simulink library "xpcmeasurementcomputinglib"  (Simulink 6.0)
settings: Solver=ode45  SolverMode=SingleTasking  StartTime=0.0  StopTime=10.0  RelTol=1e-3
undefined symbols (not defined in the file or in its folder): madcbciodas, madcbpcidas, madcbpcidas1600, mctr05checks, mdacbisa, mdacbpcidas, mdacbpcidas1600, mdacbpcidda0x12, mdiocbpcipdisox, menccbcioquadcount, misa8255, mpci8255, mtccb
libraries: xpcmeasurementcomputinglib x18
(part 4 of 4)

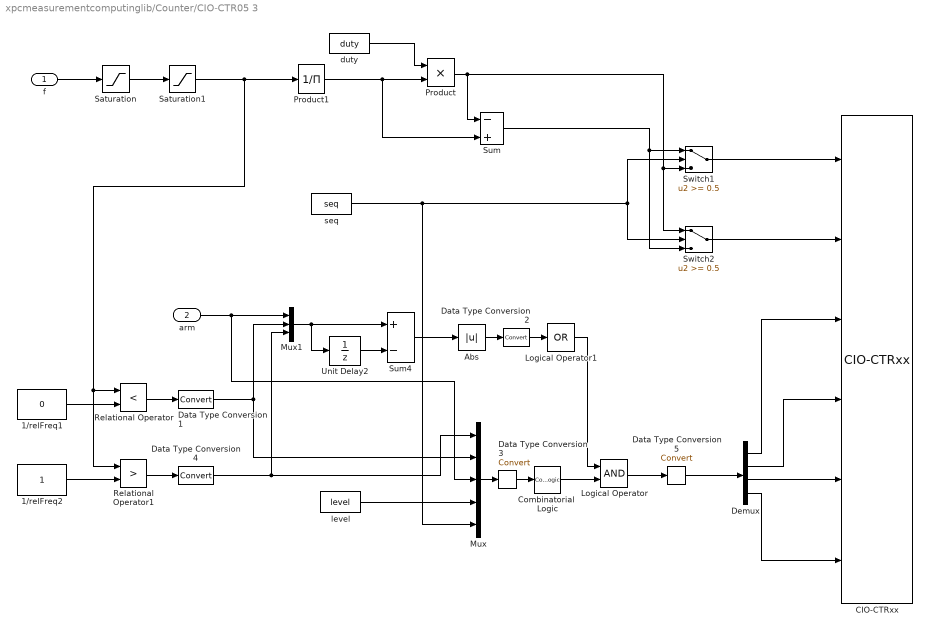
== system xpcmeasurementcomputinglib/Counter/CIO-CTR05 3 ==
  f : Inport  LatchInput=off
  arm : Inport  Port=2  LatchInput=off
  1/relFreq1 : Constant  Value=0
  1/relFreq2 : Constant
  Abs : Abs  SaturateOnIntegerOverflow=on
  "CIO-CTRxx " : xpcmeasurementcomputinglib/Counter/CIO-CTRxx   mastermode=MasterMode  countermode=CounterMode  init=Init  commands=Runtime  term=Term  ts=Ts  baseAddress=baseAddress
  Combinatorial  Logic : CombinatorialLogic  TruthTable=[0,0,1,0;0,0,1,0;0,0,0,1;0,0,0,1;0,1,0,0;1,0,0,0;0,1,0,0;1,0,0,0;0,0,1,0;0,0,1,0;0,0,0,1;0,0,0,1;0,0,1,0;0,0,1,0;0,0,1,0;0,0,1,0;0,0,1,0;0,0,1,0;0,0,0,1;0,0,0,1;0,0,0,1;0,0,0,1;0,0,0,1;0,0,0,1;0,0,0,0;0,0,0,0;0,0,0,0;0,0,0,0;0,0,0,0;0,0,0,0;0,0,0,0;0,0,0,0]
  Data Type Conversion1 : DataTypeConversion  OutDataTypeMode=double  SaturateOnIntegerOverflow=on  RndMeth=Zero
  Data Type Conversion2 : DataTypeConversion  SaturateOnIntegerOverflow=on  RndMeth=Zero
  Data Type Conversion3 : DataTypeConversion  SaturateOnIntegerOverflow=on  RndMeth=Zero
  Data Type Conversion4 : DataTypeConversion  OutDataTypeMode=double  SaturateOnIntegerOverflow=on  RndMeth=Zero
  Data Type Conversion5 : DataTypeConversion  SaturateOnIntegerOverflow=on  RndMeth=Zero
  Demux : Demux
  Logical Operator : Logic
  Logical Operator1 : Logic  Operator=OR  Inputs=1
  Mux : Mux  Inputs=5
  Mux1 : Mux  Inputs=3
  Product : Product  SaturateOnIntegerOverflow=on  InputSameDT=on
  Product1 : Product  Inputs=/  SaturateOnIntegerOverflow=on  InputSameDT=on
  Relational Operator : RelationalOperator  Operator=<  InputSameDT=on
  Relational Operator1 : RelationalOperator  Operator=>  InputSameDT=on
  Saturation : Saturate  UpperLimit=duty/2  LowerLimit=duty/(2^16-1)  ZeroCross=off
  Saturation1 : Saturate  UpperLimit=(1-duty)/2  LowerLimit=(1-duty)/(2^16-1)  ZeroCross=off
  Sum : Sum  Inputs=-+  SaturateOnIntegerOverflow=on  InputSameDT=on
  Sum4 : Sum  Inputs=+-  SaturateOnIntegerOverflow=on  InputSameDT=on
  Switch1 : Switch  Threshold=0.5  InputSameDT=on
  Switch2 : Switch  Threshold=0.5  InputSameDT=on
  Unit Delay2 : UnitDelay  X0=2  SampleTime=Ts
  duty : Constant  Value=duty
  level : Constant  Value=level
  seq : Constant  Value=seq
  wires:
  Data Type Conversion5/1 -> Demux/1
  Data Type Conversion3/1 -> Combinatorial  Logic/1
  Data Type Conversion2/1 -> Logical Operator1/1
  Data Type Conversion1/1 -> Mux1/2, Mux/2
  Data Type Conversion4/1 -> Mux1/3, Mux/1
  1/relFreq1/1 -> Relational Operator/2
  Product/1 -> Sum/1, Switch1/3, Switch2/1
  1/relFreq2/1 -> Relational Operator1/2
  Relational Operator1/1 -> Data Type Conversion4/1
  Relational Operator/1 -> Data Type Conversion1/1
  Combinatorial  Logic/1 -> Logical Operator/2
  Logical Operator/1 -> Data Type Conversion5/1
  Unit Delay2/1 -> Sum4/2
  Sum4/1 -> Abs/1
  Logical Operator1/1 -> Logical Operator/1
  Demux/1 -> "CIO-CTRxx "/3
  Demux/2 -> "CIO-CTRxx "/4
  Demux/3 -> "CIO-CTRxx "/5
  Demux/4 -> "CIO-CTRxx "/6
  level/1 -> Mux/4
  Switch1/1 -> "CIO-CTRxx "/1
  Switch2/1 -> "CIO-CTRxx "/2
  seq/1 -> Switch1/2, Switch2/2, Mux/5
  Sum/1 -> Switch1/1, Switch2/3
  Saturation/1 -> Saturation1/1
  f/1 -> Saturation/1
  Mux1/1 -> Sum4/1, Unit Delay2/1
  arm/1 -> Mux1/1, Mux/3
  Abs/1 -> Data Type Conversion2/1
  Mux/1 -> Data Type Conversion3/1
  Saturation1/1 -> Product1/1, Relational Operator1/1, Relational Operator/1
  duty/1 -> Product/1
  Product1/1 -> Product/2, Sum/2

== system xpcmeasurementcomputinglib/Counter/CIO-CTR05 4 ==
  "CIO-CTRxx " : xpcmeasurementcomputinglib/Counter/CIO-CTRxx   mastermode=MasterMode  countermode=CounterMode  init=Init  commands=Runtime  term=Term  ts=Ts  baseAddress=baseAddress
  Demux : Demux  Outputs=2
  Product : Product  Inputs=/  SaturateOnIntegerOverflow=on  InputSameDT=on
  Product1 : Product  Inputs=**  SaturateOnIntegerOverflow=on  InputSameDT=on
  f : Outport
  dc : Outport  Port=2
  wires:
  Product1/1 -> dc/1
  Product/1 -> Product1/2, f/1
  Demux/2 -> Product/1
  Demux/1 -> Product1/1
  "CIO-CTRxx "/1 -> Demux/1

== system xpcmeasurementcomputinglib/Counter/CIO-CTR05 5 ==
  "CIO-CTRxx " : xpcmeasurementcomputinglib/Counter/CIO-CTRxx   mastermode=MasterMode  countermode=CounterMode  init=Init  commands=Runtime  term=Term  ts=Ts  baseAddress=baseAddress
  Product : Product  Inputs=/  SaturateOnIntegerOverflow=on  InputSameDT=on
  f : Outport
  wires:
  Product/1 -> f/1
  "CIO-CTRxx "/1 -> Product/1

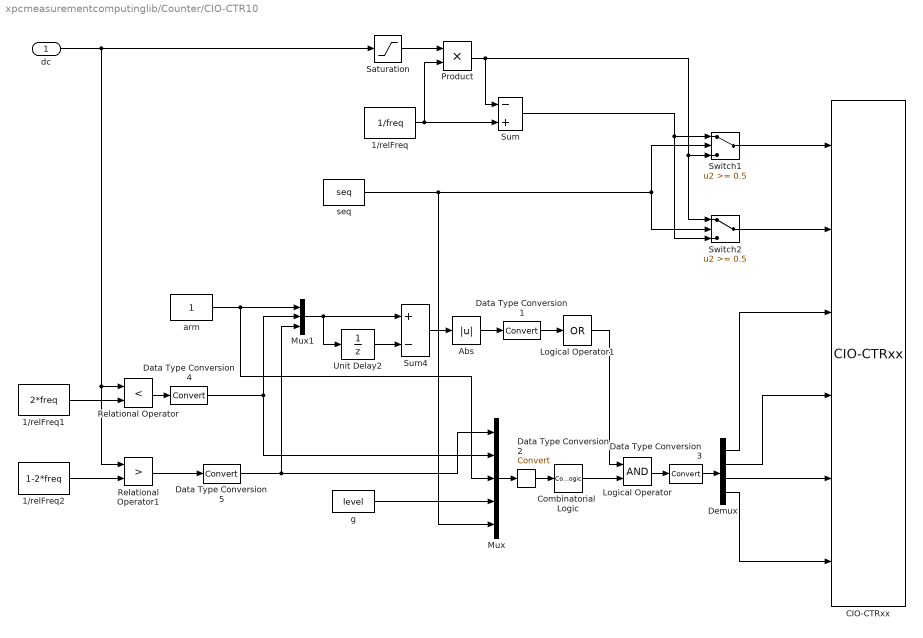
== system xpcmeasurementcomputinglib/Counter/CIO-CTR10  ==
  dc : Inport  LatchInput=off
  1/relFreq : Constant  Value=1/freq
  1/relFreq1 : Constant  Value=2*freq
  1/relFreq2 : Constant  Value=1-2*freq
  Abs : Abs  SaturateOnIntegerOverflow=on
  "CIO-CTRxx " : xpcmeasurementcomputinglib/Counter/CIO-CTRxx   mastermode=MasterMode  countermode=CounterMode  init=Init  commands=Runtime  term=Term  ts=Ts  baseAddress=baseAddress
  Combinatorial  Logic : CombinatorialLogic  TruthTable=[0,0,1,0;0,0,1,0;0,0,0,1;0,0,0,1;0,1,0,0;1,0,0,0;0,1,0,0;1,0,0,0;0,0,1,0;0,0,1,0;0,0,0,1;0,0,0,1;0,0,1,0;0,0,1,0;0,0,1,0;0,0,1,0;0,0,1,0;0,0,1,0;0,0,0,1;0,0,0,1;0,0,0,1;0,0,0,1;0,0,0,1;0,0,0,1;0,0,0,0;0,0,0,0;0,0,0,0;0,0,0,0;0,0,0,0;0,0,0,0;0,0,0,0;0,0,0,0]
  Data Type Conversion1 : DataTypeConversion  SaturateOnIntegerOverflow=on  RndMeth=Zero
  Data Type Conversion2 : DataTypeConversion  SaturateOnIntegerOverflow=on  RndMeth=Zero
  Data Type Conversion3 : DataTypeConversion  SaturateOnIntegerOverflow=on  RndMeth=Zero
  Data Type Conversion4 : DataTypeConversion  OutDataTypeMode=double  SaturateOnIntegerOverflow=on  RndMeth=Zero
  Data Type Conversion5 : DataTypeConversion  OutDataTypeMode=double  SaturateOnIntegerOverflow=on  RndMeth=Zero
  Demux : Demux
  Logical Operator : Logic
  Logical Operator1 : Logic  Operator=OR  Inputs=1
  Mux : Mux  Inputs=5
  Mux1 : Mux  Inputs=3
  Product : Product  SaturateOnIntegerOverflow=on  InputSameDT=on
  Relational Operator : RelationalOperator  Operator=<  InputSameDT=on
  Relational Operator1 : RelationalOperator  Operator=>  InputSameDT=on
  Saturation : Saturate  UpperLimit=1-2*freq  LowerLimit=2*freq  ZeroCross=off
  Sum : Sum  Inputs=-+  SaturateOnIntegerOverflow=on  InputSameDT=on
  Sum4 : Sum  Inputs=+-  SaturateOnIntegerOverflow=on  InputSameDT=on
  Switch1 : Switch  Threshold=0.5  InputSameDT=on
  Switch2 : Switch  Threshold=0.5  InputSameDT=on
  Unit Delay2 : UnitDelay  X0=2  SampleTime=Ts
  arm : Constant
  g : Constant  Value=level
  seq : Constant  Value=seq
  wires:
  Data Type Conversion5/1 -> Mux1/3, Mux/1
  Data Type Conversion4/1 -> Mux1/2, Mux/2
  Data Type Conversion3/1 -> Demux/1
  Data Type Conversion2/1 -> Combinatorial  Logic/1
  Data Type Conversion1/1 -> Logical Operator1/1
  1/relFreq1/1 -> Relational Operator/2
  1/relFreq/1 -> Product/2, Sum/2
  Product/1 -> Sum/1, Switch1/3, Switch2/1
  1/relFreq2/1 -> Relational Operator1/2
  Relational Operator1/1 -> Data Type Conversion5/1
  Relational Operator/1 -> Data Type Conversion4/1
  Combinatorial  Logic/1 -> Logical Operator/2
  Logical Operator/1 -> Data Type Conversion3/1
  Unit Delay2/1 -> Sum4/2
  Sum4/1 -> Abs/1
  Logical Operator1/1 -> Logical Operator/1
  Demux/1 -> "CIO-CTRxx "/3
  Demux/2 -> "CIO-CTRxx "/4
  Demux/3 -> "CIO-CTRxx "/5
  Demux/4 -> "CIO-CTRxx "/6
  g/1 -> Mux/4
  seq/1 -> Switch1/2, Switch2/2, Mux/5
  Sum/1 -> Switch1/1, Switch2/3
  Saturation/1 -> Product/1
  dc/1 -> Saturation/1, Relational Operator/1, Relational Operator1/1
  Mux1/1 -> Sum4/1, Unit Delay2/1
  arm/1 -> Mux1/1, Mux/3
  Abs/1 -> Data Type Conversion1/1
  Mux/1 -> Data Type Conversion2/1
  Switch1/1 -> "CIO-CTRxx "/1
  Switch2/1 -> "CIO-CTRxx "/2

== system xpcmeasurementcomputinglib/Counter/CIO-CTR10 1 ==
  dc : Inport  LatchInput=off
  arm : Inport  Port=2  LatchInput=off
  1/relFreq : Constant  Value=1/freq
  1/relFreq1 : Constant  Value=2*freq
  1/relFreq2 : Constant  Value=1-2*freq
  Abs : Abs  SaturateOnIntegerOverflow=on
  "CIO-CTRxx " : xpcmeasurementcomputinglib/Counter/CIO-CTRxx   mastermode=MasterMode  countermode=CounterMode  init=Init  commands=Runtime  term=Term  ts=Ts  baseAddress=baseAddress
  Combinatorial  Logic : CombinatorialLogic  TruthTable=[0,0,1,0;0,0,1,0;0,0,0,1;0,0,0,1;0,1,0,0;1,0,0,0;0,1,0,0;1,0,0,0;0,0,1,0;0,0,1,0;0,0,0,1;0,0,0,1;0,0,1,0;0,0,1,0;0,0,1,0;0,0,1,0;0,0,1,0;0,0,1,0;0,0,0,1;0,0,0,1;0,0,0,1;0,0,0,1;0,0,0,1;0,0,0,1;0,0,0,0;0,0,0,0;0,0,0,0;0,0,0,0;0,0,0,0;0,0,0,0;0,0,0,0;0,0,0,0]
  Data Type Conversion1 : DataTypeConversion  SaturateOnIntegerOverflow=on  RndMeth=Zero
  Data Type Conversion2 : DataTypeConversion  SaturateOnIntegerOverflow=on  RndMeth=Zero
  Data Type Conversion3 : DataTypeConversion  SaturateOnIntegerOverflow=on  RndMeth=Zero
  Data Type Conversion4 : DataTypeConversion  OutDataTypeMode=double  SaturateOnIntegerOverflow=on  RndMeth=Zero
  Data Type Conversion5 : DataTypeConversion  OutDataTypeMode=double  SaturateOnIntegerOverflow=on  RndMeth=Zero
  Demux : Demux
  Logical Operator : Logic
  Logical Operator1 : Logic  Operator=OR  Inputs=1
  Mux : Mux  Inputs=5
  Mux1 : Mux  Inputs=3
  Product : Product  SaturateOnIntegerOverflow=on  InputSameDT=on
  Relational Operator : RelationalOperator  Operator=<  InputSameDT=on
  Relational Operator1 : RelationalOperator  Operator=>  InputSameDT=on
  Saturation : Saturate  UpperLimit=1-2*freq  LowerLimit=2*freq  ZeroCross=off
  Sum : Sum  Inputs=-+  SaturateOnIntegerOverflow=on  InputSameDT=on
  Sum4 : Sum  Inputs=+-  SaturateOnIntegerOverflow=on  InputSameDT=on
  Switch1 : Switch  Threshold=0.5  InputSameDT=on
  Switch2 : Switch  Threshold=0.5  InputSameDT=on
  Unit Delay2 : UnitDelay  X0=2  SampleTime=Ts
  g : Constant  Value=level
  seq : Constant  Value=seq
  wires:
  Data Type Conversion5/1 -> Mux1/3, Mux/1
  Data Type Conversion4/1 -> Mux1/2, Mux/2
  Data Type Conversion3/1 -> Combinatorial  Logic/1
  Data Type Conversion2/1 -> Logical Operator1/1
  Data Type Conversion1/1 -> Demux/1
  1/relFreq1/1 -> Relational Operator/2
  1/relFreq/1 -> Product/2, Sum/2
  Product/1 -> Sum/1, Switch1/3, Switch2/1
  1/relFreq2/1 -> Relational Operator1/2
  Relational Operator1/1 -> Data Type Conversion5/1
  Relational Operator/1 -> Data Type Conversion4/1
  Combinatorial  Logic/1 -> Logical Operator/2
  Logical Operator/1 -> Data Type Conversion1/1
  Unit Delay2/1 -> Sum4/2
  Sum4/1 -> Abs/1
  Logical Operator1/1 -> Logical Operator/1
  Demux/1 -> "CIO-CTRxx "/3
  Demux/2 -> "CIO-CTRxx "/4
  Demux/3 -> "CIO-CTRxx "/5
  Demux/4 -> "CIO-CTRxx "/6
  g/1 -> Mux/4
  seq/1 -> Switch1/2, Switch2/2, Mux/5
  Sum/1 -> Switch1/1, Switch2/3
  Saturation/1 -> Product/1
  dc/1 -> Saturation/1, Relational Operator/1, Relational Operator1/1
  Mux1/1 -> Sum4/1, Unit Delay2/1
  arm/1 -> Mux1/1, Mux/3
  Abs/1 -> Data Type Conversion2/1
  Mux/1 -> Data Type Conversion3/1
  Switch1/1 -> "CIO-CTRxx "/1
  Switch2/1 -> "CIO-CTRxx "/2

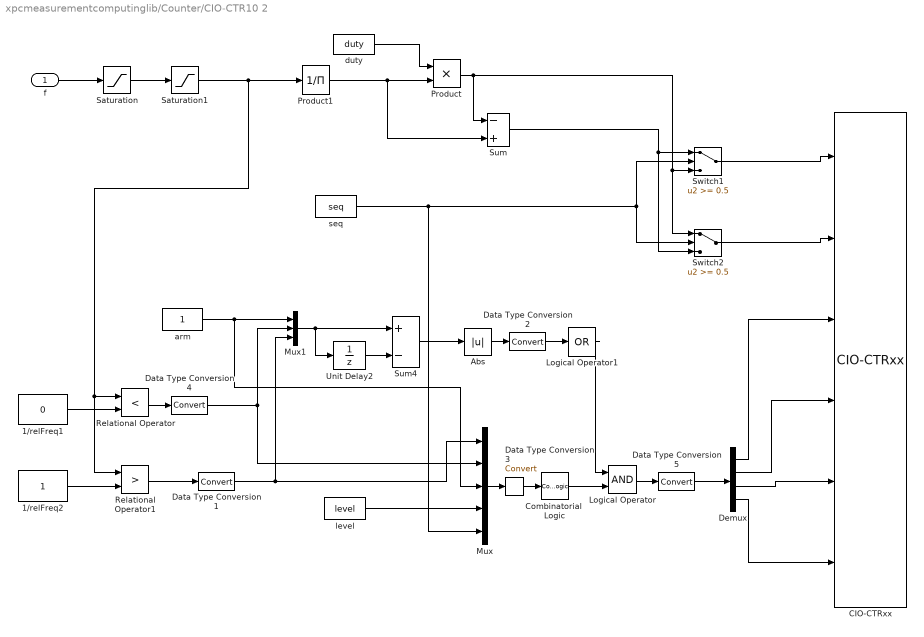
== system xpcmeasurementcomputinglib/Counter/CIO-CTR10 2 ==
  f : Inport  LatchInput=off
  1/relFreq1 : Constant  Value=0
  1/relFreq2 : Constant
  Abs : Abs  SaturateOnIntegerOverflow=on
  "CIO-CTRxx " : xpcmeasurementcomputinglib/Counter/CIO-CTRxx   mastermode=MasterMode  countermode=CounterMode  init=Init  commands=Runtime  term=Term  ts=Ts  baseAddress=baseAddress
  Combinatorial  Logic : CombinatorialLogic  TruthTable=[0,0,1,0;0,0,1,0;0,0,0,1;0,0,0,1;0,1,0,0;1,0,0,0;0,1,0,0;1,0,0,0;0,0,1,0;0,0,1,0;0,0,0,1;0,0,0,1;0,0,1,0;0,0,1,0;0,0,1,0;0,0,1,0;0,0,1,0;0,0,1,0;0,0,0,1;0,0,0,1;0,0,0,1;0,0,0,1;0,0,0,1;0,0,0,1;0,0,0,0;0,0,0,0;0,0,0,0;0,0,0,0;0,0,0,0;0,0,0,0;0,0,0,0;0,0,0,0]
  Data Type Conversion1 : DataTypeConversion  OutDataTypeMode=double  SaturateOnIntegerOverflow=on  RndMeth=Zero
  Data Type Conversion2 : DataTypeConversion  SaturateOnIntegerOverflow=on  RndMeth=Zero
  Data Type Conversion3 : DataTypeConversion  SaturateOnIntegerOverflow=on  RndMeth=Zero
  Data Type Conversion4 : DataTypeConversion  OutDataTypeMode=double  SaturateOnIntegerOverflow=on  RndMeth=Zero
  Data Type Conversion5 : DataTypeConversion  SaturateOnIntegerOverflow=on  RndMeth=Zero
  Demux : Demux
  Logical Operator : Logic
  Logical Operator1 : Logic  Operator=OR  Inputs=1
  Mux : Mux  Inputs=5
  Mux1 : Mux  Inputs=3
  Product : Product  SaturateOnIntegerOverflow=on  InputSameDT=on
  Product1 : Product  Inputs=/  SaturateOnIntegerOverflow=on  InputSameDT=on
  Relational Operator : RelationalOperator  Operator=<  InputSameDT=on
  Relational Operator1 : RelationalOperator  Operator=>  InputSameDT=on
  Saturation : Saturate  UpperLimit=duty/2  LowerLimit=duty/(2^16-1)  ZeroCross=off
  Saturation1 : Saturate  UpperLimit=(1-duty)/2  LowerLimit=(1-duty)/(2^16-1)  ZeroCross=off
  Sum : Sum  Inputs=-+  SaturateOnIntegerOverflow=on  InputSameDT=on
  Sum4 : Sum  Inputs=+-  SaturateOnIntegerOverflow=on  InputSameDT=on
  Switch1 : Switch  Threshold=0.5  InputSameDT=on
  Switch2 : Switch  Threshold=0.5  InputSameDT=on
  Unit Delay2 : UnitDelay  X0=2  SampleTime=Ts
  arm : Constant
  duty : Constant  Value=duty
  level : Constant  Value=level
  seq : Constant  Value=seq
  wires:
  Data Type Conversion5/1 -> Demux/1
  Data Type Conversion3/1 -> Combinatorial  Logic/1
  Data Type Conversion2/1 -> Logical Operator1/1
  Data Type Conversion1/1 -> Mux1/3, Mux/1
  Data Type Conversion4/1 -> Mux1/2, Mux/2
  1/relFreq1/1 -> Relational Operator/2
  Product/1 -> Sum/1, Switch1/3, Switch2/1
  1/relFreq2/1 -> Relational Operator1/2
  Relational Operator1/1 -> Data Type Conversion1/1
  Relational Operator/1 -> Data Type Conversion4/1
  Combinatorial  Logic/1 -> Logical Operator/2
  Logical Operator/1 -> Data Type Conversion5/1
  Unit Delay2/1 -> Sum4/2
  Sum4/1 -> Abs/1
  Logical Operator1/1 -> Logical Operator/1
  Demux/1 -> "CIO-CTRxx "/3
  Demux/2 -> "CIO-CTRxx "/4
  Demux/3 -> "CIO-CTRxx "/5
  Demux/4 -> "CIO-CTRxx "/6
  level/1 -> Mux/4
  Switch1/1 -> "CIO-CTRxx "/1
  Switch2/1 -> "CIO-CTRxx "/2
  seq/1 -> Switch1/2, Switch2/2, Mux/5
  Sum/1 -> Switch1/1, Switch2/3
  Saturation/1 -> Saturation1/1
  f/1 -> Saturation/1
  Mux1/1 -> Sum4/1, Unit Delay2/1
  arm/1 -> Mux1/1, Mux/3
  Abs/1 -> Data Type Conversion2/1
  Mux/1 -> Data Type Conversion3/1
  Saturation1/1 -> Product1/1, Relational Operator1/1, Relational Operator/1
  duty/1 -> Product/1
  Product1/1 -> Product/2, Sum/2

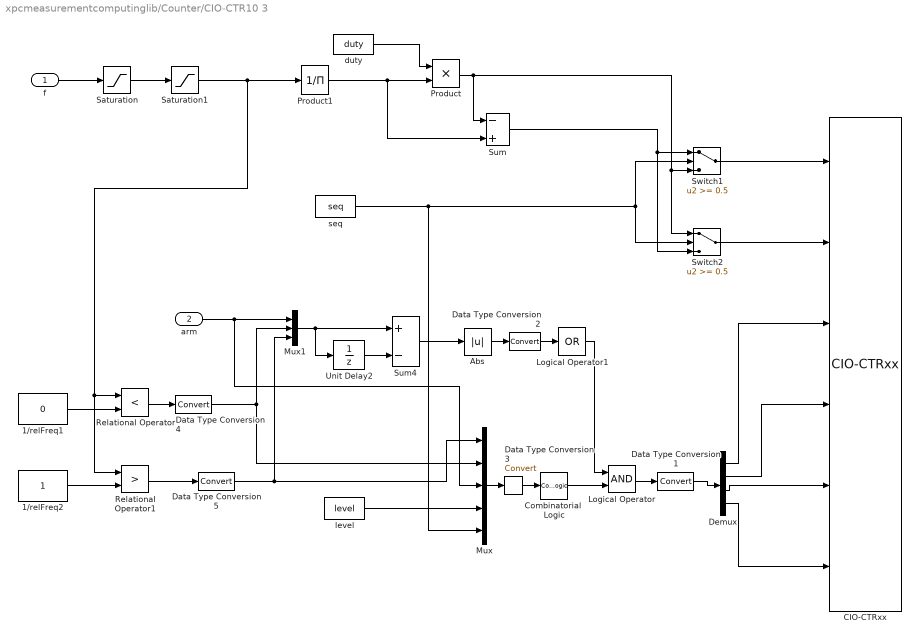
== system xpcmeasurementcomputinglib/Counter/CIO-CTR10 3 ==
  f : Inport  LatchInput=off
  arm : Inport  Port=2  LatchInput=off
  1/relFreq1 : Constant  Value=0
  1/relFreq2 : Constant
  Abs : Abs  SaturateOnIntegerOverflow=on
  "CIO-CTRxx " : xpcmeasurementcomputinglib/Counter/CIO-CTRxx   mastermode=MasterMode  countermode=CounterMode  init=Init  commands=Runtime  term=Term  ts=Ts  baseAddress=baseAddress
  Combinatorial  Logic : CombinatorialLogic  TruthTable=[0,0,1,0;0,0,1,0;0,0,0,1;0,0,0,1;0,1,0,0;1,0,0,0;0,1,0,0;1,0,0,0;0,0,1,0;0,0,1,0;0,0,0,1;0,0,0,1;0,0,1,0;0,0,1,0;0,0,1,0;0,0,1,0;0,0,1,0;0,0,1,0;0,0,0,1;0,0,0,1;0,0,0,1;0,0,0,1;0,0,0,1;0,0,0,1;0,0,0,0;0,0,0,0;0,0,0,0;0,0,0,0;0,0,0,0;0,0,0,0;0,0,0,0;0,0,0,0]
  Data Type Conversion1 : DataTypeConversion  SaturateOnIntegerOverflow=on  RndMeth=Zero
  Data Type Conversion2 : DataTypeConversion  SaturateOnIntegerOverflow=on  RndMeth=Zero
  Data Type Conversion3 : DataTypeConversion  SaturateOnIntegerOverflow=on  RndMeth=Zero
  Data Type Conversion4 : DataTypeConversion  OutDataTypeMode=double  SaturateOnIntegerOverflow=on  RndMeth=Zero
  Data Type Conversion5 : DataTypeConversion  OutDataTypeMode=double  SaturateOnIntegerOverflow=on  RndMeth=Zero
  Demux : Demux
  Logical Operator : Logic
  Logical Operator1 : Logic  Operator=OR  Inputs=1
  Mux : Mux  Inputs=5
  Mux1 : Mux  Inputs=3
  Product : Product  SaturateOnIntegerOverflow=on  InputSameDT=on
  Product1 : Product  Inputs=/  SaturateOnIntegerOverflow=on  InputSameDT=on
  Relational Operator : RelationalOperator  Operator=<  InputSameDT=on
  Relational Operator1 : RelationalOperator  Operator=>  InputSameDT=on
  Saturation : Saturate  UpperLimit=duty/2  LowerLimit=duty/(2^16-1)  ZeroCross=off
  Saturation1 : Saturate  UpperLimit=(1-duty)/2  LowerLimit=(1-duty)/(2^16-1)  ZeroCross=off
  Sum : Sum  Inputs=-+  SaturateOnIntegerOverflow=on  InputSameDT=on
  Sum4 : Sum  Inputs=+-  SaturateOnIntegerOverflow=on  InputSameDT=on
  Switch1 : Switch  Threshold=0.5  InputSameDT=on
  Switch2 : Switch  Threshold=0.5  InputSameDT=on
  Unit Delay2 : UnitDelay  X0=2  SampleTime=Ts
  duty : Constant  Value=duty
  level : Constant  Value=level
  seq : Constant  Value=seq
  wires:
  Data Type Conversion5/1 -> Mux1/3, Mux/1
  Data Type Conversion4/1 -> Mux1/2, Mux/2
  Data Type Conversion3/1 -> Combinatorial  Logic/1
  Data Type Conversion2/1 -> Logical Operator1/1
  Data Type Conversion1/1 -> Demux/1
  1/relFreq1/1 -> Relational Operator/2
  Product/1 -> Sum/1, Switch1/3, Switch2/1
  1/relFreq2/1 -> Relational Operator1/2
  Relational Operator1/1 -> Data Type Conversion5/1
  Relational Operator/1 -> Data Type Conversion4/1
  Combinatorial  Logic/1 -> Logical Operator/2
  Logical Operator/1 -> Data Type Conversion1/1
  Unit Delay2/1 -> Sum4/2
  Sum4/1 -> Abs/1
  Logical Operator1/1 -> Logical Operator/1
  Demux/1 -> "CIO-CTRxx "/3
  Demux/2 -> "CIO-CTRxx "/4
  Demux/3 -> "CIO-CTRxx "/5
  Demux/4 -> "CIO-CTRxx "/6
  level/1 -> Mux/4
  Switch1/1 -> "CIO-CTRxx "/1
  Switch2/1 -> "CIO-CTRxx "/2
  seq/1 -> Switch1/2, Switch2/2, Mux/5
  Sum/1 -> Switch1/1, Switch2/3
  Saturation/1 -> Saturation1/1
  f/1 -> Saturation/1
  Mux1/1 -> Sum4/1, Unit Delay2/1
  arm/1 -> Mux1/1, Mux/3
  Abs/1 -> Data Type Conversion2/1
  Mux/1 -> Data Type Conversion3/1
  Saturation1/1 -> Product1/1, Relational Operator1/1, Relational Operator/1
  duty/1 -> Product/1
  Product1/1 -> Product/2, Sum/2

== system xpcmeasurementcomputinglib/Counter/CIO-CTR10 4 ==
  "CIO-CTRxx " : xpcmeasurementcomputinglib/Counter/CIO-CTRxx   mastermode=MasterMode  countermode=CounterMode  init=Init  commands=Runtime  term=Term  ts=Ts  baseAddress=baseAddress
  Demux : Demux  Outputs=2
  Product : Product  Inputs=/  SaturateOnIntegerOverflow=on  InputSameDT=on
  Product1 : Product  Inputs=**  SaturateOnIntegerOverflow=on  InputSameDT=on
  f : Outport
  dc : Outport  Port=2
  wires:
  Product1/1 -> dc/1
  Product/1 -> Product1/2, f/1
  Demux/2 -> Product/1
  Demux/1 -> Product1/1
  "CIO-CTRxx "/1 -> Demux/1

== system xpcmeasurementcomputinglib/Counter/CIO-CTR10 5 ==
  "CIO-CTRxx " : xpcmeasurementcomputinglib/Counter/CIO-CTRxx   mastermode=MasterMode  countermode=CounterMode  init=Init  commands=Runtime  term=Term  ts=Ts  baseAddress=baseAddress
  Product : Product  Inputs=/  SaturateOnIntegerOverflow=on  InputSameDT=on
  f : Outport
  wires:
  Product/1 -> f/1
  "CIO-CTRxx "/1 -> Product/1

== system xpcmeasurementcomputinglib/Counter/PCI-CTR05  ==
  dc : Inport  LatchInput=off
  1/relFreq : Constant  Value=1/freq
  1/relFreq1 : Constant  Value=2*freq
  1/relFreq2 : Constant  Value=1-2*freq
  Abs : Abs  SaturateOnIntegerOverflow=on
  Combinatorial  Logic : CombinatorialLogic  TruthTable=[0,0,1,0;0,0,1,0;0,0,0,1;0,0,0,1;0,1,0,0;1,0,0,0;0,1,0,0;1,0,0,0;0,0,1,0;0,0,1,0;0,0,0,1;0,0,0,1;0,0,1,0;0,0,1,0;0,0,1,0;0,0,1,0;0,0,1,0;0,0,1,0;0,0,0,1;0,0,0,1;0,0,0,1;0,0,0,1;0,0,0,1;0,0,0,1;0,0,0,0;0,0,0,0;0,0,0,0;0,0,0,0;0,0,0,0;0,0,0,0;0,0,0,0;0,0,0,0]
  Data Type Conversion1 : DataTypeConversion  OutDataTypeMode=double  SaturateOnIntegerOverflow=on  RndMeth=Zero
  Data Type Conversion2 : DataTypeConversion  SaturateOnIntegerOverflow=on  RndMeth=Zero
  Data Type Conversion3 : DataTypeConversion  SaturateOnIntegerOverflow=on  RndMeth=Zero
  Data Type Conversion4 : DataTypeConversion  OutDataTypeMode=double  SaturateOnIntegerOverflow=on  RndMeth=Zero
  Data Type Conversion5 : DataTypeConversion  SaturateOnIntegerOverflow=on  RndMeth=Zero
  Demux : Demux
  Logical Operator : Logic
  Logical Operator1 : Logic  Operator=OR  Inputs=1
  Mux : Mux  Inputs=5
  Mux1 : Mux  Inputs=3
  "PCI-CTR05  " : xpcmeasurementcomputinglib/Counter/PCI-CTR05    mastermode=MasterMode  countermode=CounterMode  init=Init  commands=Runtime  term=Term  ts=Ts  pciSlot=pciSlot
  Product : Product  SaturateOnIntegerOverflow=on  InputSameDT=on
  Relational Operator : RelationalOperator  Operator=<  InputSameDT=on
  Relational Operator1 : RelationalOperator  Operator=>  InputSameDT=on
  Saturation : Saturate  UpperLimit=1-2*freq  LowerLimit=2*freq  ZeroCross=off
  Sum : Sum  Inputs=-+  SaturateOnIntegerOverflow=on  InputSameDT=on
  Sum4 : Sum  Inputs=+-  SaturateOnIntegerOverflow=on  InputSameDT=on
  Switch1 : Switch  Threshold=0.5  InputSameDT=on
  Switch2 : Switch  Threshold=0.5  InputSameDT=on
  Unit Delay2 : UnitDelay  X0=2  SampleTime=Ts
  arm : Constant
  level : Constant  Value=level
  seq : Constant  Value=seq
  wires:
  Data Type Conversion5/1 -> Demux/1
  Data Type Conversion3/1 -> Combinatorial  Logic/1
  Data Type Conversion2/1 -> Logical Operator1/1
  Data Type Conversion1/1 -> Mux1/2, Mux/2
  Data Type Conversion4/1 -> Mux1/3, Mux/1
  1/relFreq1/1 -> Relational Operator/2
  1/relFreq/1 -> Product/2, Sum/2
  Product/1 -> Sum/1, Switch1/3, Switch2/1
  1/relFreq2/1 -> Relational Operator1/2
  Relational Operator1/1 -> Data Type Conversion4/1
  Relational Operator/1 -> Data Type Conversion1/1
  Combinatorial  Logic/1 -> Logical Operator/2
  Logical Operator/1 -> Data Type Conversion5/1
  Unit Delay2/1 -> Sum4/2
  Sum4/1 -> Abs/1
  Logical Operator1/1 -> Logical Operator/1
  Demux/1 -> "PCI-CTR05  "/3
  Demux/2 -> "PCI-CTR05  "/4
  Demux/3 -> "PCI-CTR05  "/5
  Demux/4 -> "PCI-CTR05  "/6
  level/1 -> Mux/4
  Switch1/1 -> "PCI-CTR05  "/1
  Switch2/1 -> "PCI-CTR05  "/2
  seq/1 -> Switch1/2, Switch2/2, Mux/5
  Sum/1 -> Switch1/1, Switch2/3
  Saturation/1 -> Product/1
  dc/1 -> Saturation/1, Relational Operator/1, Relational Operator1/1
  Mux1/1 -> Sum4/1, Unit Delay2/1
  arm/1 -> Mux1/1, Mux/3
  Abs/1 -> Data Type Conversion2/1
  Mux/1 -> Data Type Conversion3/1

== system xpcmeasurementcomputinglib/Counter/PCI-CTR05 1 ==
  dc : Inport  LatchInput=off
  arm : Inport  Port=2  LatchInput=off
  1/relFreq : Constant  Value=1/freq
  1/relFreq1 : Constant  Value=2*freq
  1/relFreq2 : Constant  Value=1-2*freq
  Abs : Abs  SaturateOnIntegerOverflow=on
  Combinatorial  Logic : CombinatorialLogic  TruthTable=[0,0,1,0;0,0,1,0;0,0,0,1;0,0,0,1;0,1,0,0;1,0,0,0;0,1,0,0;1,0,0,0;0,0,1,0;0,0,1,0;0,0,0,1;0,0,0,1;0,0,1,0;0,0,1,0;0,0,1,0;0,0,1,0;0,0,1,0;0,0,1,0;0,0,0,1;0,0,0,1;0,0,0,1;0,0,0,1;0,0,0,1;0,0,0,1;0,0,0,0;0,0,0,0;0,0,0,0;0,0,0,0;0,0,0,0;0,0,0,0;0,0,0,0;0,0,0,0]
  Data Type Conversion1 : DataTypeConversion  OutDataTypeMode=double  SaturateOnIntegerOverflow=on  RndMeth=Zero
  Data Type Conversion2 : DataTypeConversion  SaturateOnIntegerOverflow=on  RndMeth=Zero
  Data Type Conversion3 : DataTypeConversion  SaturateOnIntegerOverflow=on  RndMeth=Zero
  Data Type Conversion4 : DataTypeConversion  OutDataTypeMode=double  SaturateOnIntegerOverflow=on  RndMeth=Zero
  Data Type Conversion5 : DataTypeConversion  SaturateOnIntegerOverflow=on  RndMeth=Zero
  Demux : Demux
  Logical Operator : Logic
  Logical Operator1 : Logic  Operator=OR  Inputs=1
  Mux : Mux  Inputs=5
  Mux1 : Mux  Inputs=3
  "PCI-CTR05  " : xpcmeasurementcomputinglib/Counter/PCI-CTR05    mastermode=MasterMode  countermode=CounterMode  init=Init  commands=Runtime  term=Term  ts=Ts  pciSlot=pciSlot
  Product : Product  SaturateOnIntegerOverflow=on  InputSameDT=on
  Relational Operator : RelationalOperator  Operator=<  InputSameDT=on
  Relational Operator1 : RelationalOperator  Operator=>  InputSameDT=on
  Saturation : Saturate  UpperLimit=1-2*freq  LowerLimit=2*freq  ZeroCross=off
  Sum : Sum  Inputs=-+  SaturateOnIntegerOverflow=on  InputSameDT=on
  Sum4 : Sum  Inputs=+-  SaturateOnIntegerOverflow=on  InputSameDT=on
  Switch1 : Switch  Threshold=0.5  InputSameDT=on
  Switch2 : Switch  Threshold=0.5  InputSameDT=on
  Unit Delay2 : UnitDelay  X0=2  SampleTime=Ts
  level : Constant  Value=level
  seq : Constant  Value=seq
  wires:
  Data Type Conversion5/1 -> Logical Operator1/1
  Data Type Conversion3/1 -> Demux/1
  Data Type Conversion2/1 -> Combinatorial  Logic/1
  Data Type Conversion1/1 -> Mux1/3, Mux/1
  Data Type Conversion4/1 -> Mux1/2, Mux/2
  1/relFreq1/1 -> Relational Operator/2
  1/relFreq/1 -> Product/2, Sum/2
  Product/1 -> Sum/1, Switch1/3, Switch2/1
  1/relFreq2/1 -> Relational Operator1/2
  Relational Operator1/1 -> Data Type Conversion1/1
  Relational Operator/1 -> Data Type Conversion4/1
  Combinatorial  Logic/1 -> Logical Operator/2
  Logical Operator/1 -> Data Type Conversion3/1
  Unit Delay2/1 -> Sum4/2
  Sum4/1 -> Abs/1
  Logical Operator1/1 -> Logical Operator/1
  Demux/1 -> "PCI-CTR05  "/3
  Demux/2 -> "PCI-CTR05  "/4
  Demux/3 -> "PCI-CTR05  "/5
  Demux/4 -> "PCI-CTR05  "/6
  level/1 -> Mux/4
  Switch1/1 -> "PCI-CTR05  "/1
  Switch2/1 -> "PCI-CTR05  "/2
  seq/1 -> Switch1/2, Switch2/2, Mux/5
  Sum/1 -> Switch1/1, Switch2/3
  Saturation/1 -> Product/1
  dc/1 -> Saturation/1, Relational Operator/1, Relational Operator1/1
  Mux1/1 -> Sum4/1, Unit Delay2/1
  arm/1 -> Mux1/1, Mux/3
  Abs/1 -> Data Type Conversion5/1
  Mux/1 -> Data Type Conversion2/1

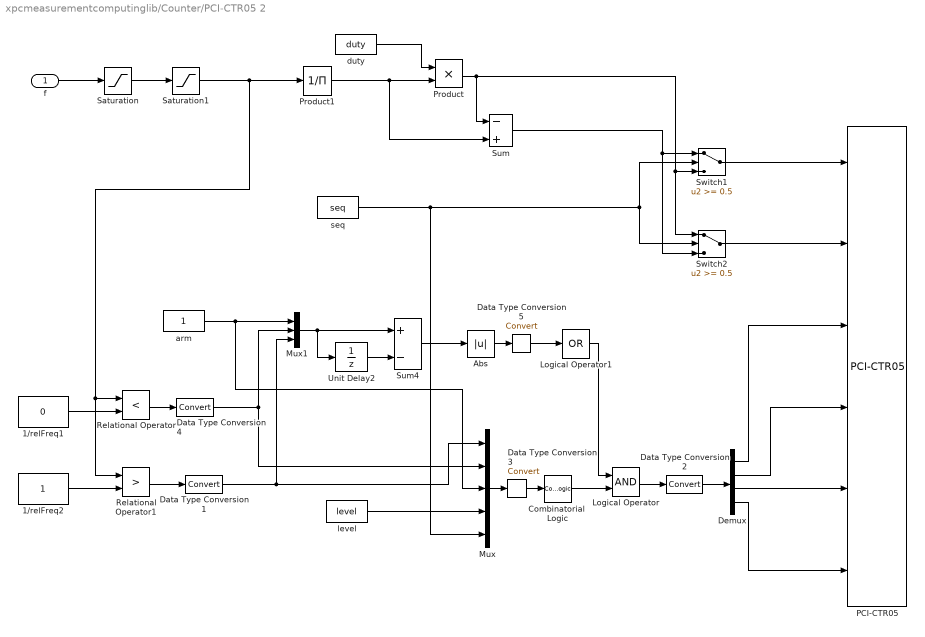
== system xpcmeasurementcomputinglib/Counter/PCI-CTR05 2 ==
  f : Inport  LatchInput=off
  1/relFreq1 : Constant  Value=0
  1/relFreq2 : Constant
  Abs : Abs  SaturateOnIntegerOverflow=on
  Combinatorial  Logic : CombinatorialLogic  TruthTable=[0,0,1,0;0,0,1,0;0,0,0,1;0,0,0,1;0,1,0,0;1,0,0,0;0,1,0,0;1,0,0,0;0,0,1,0;0,0,1,0;0,0,0,1;0,0,0,1;0,0,1,0;0,0,1,0;0,0,1,0;0,0,1,0;0,0,1,0;0,0,1,0;0,0,0,1;0,0,0,1;0,0,0,1;0,0,0,1;0,0,0,1;0,0,0,1;0,0,0,0;0,0,0,0;0,0,0,0;0,0,0,0;0,0,0,0;0,0,0,0;0,0,0,0;0,0,0,0]
  Data Type Conversion1 : DataTypeConversion  OutDataTypeMode=double  SaturateOnIntegerOverflow=on  RndMeth=Zero
  Data Type Conversion2 : DataTypeConversion  SaturateOnIntegerOverflow=on  RndMeth=Zero
  Data Type Conversion3 : DataTypeConversion  SaturateOnIntegerOverflow=on  RndMeth=Zero
  Data Type Conversion4 : DataTypeConversion  OutDataTypeMode=double  SaturateOnIntegerOverflow=on  RndMeth=Zero
  Data Type Conversion5 : DataTypeConversion  SaturateOnIntegerOverflow=on  RndMeth=Zero
  Demux : Demux
  Logical Operator : Logic
  Logical Operator1 : Logic  Operator=OR  Inputs=1
  Mux : Mux  Inputs=5
  Mux1 : Mux  Inputs=3
  "PCI-CTR05  " : xpcmeasurementcomputinglib/Counter/PCI-CTR05    mastermode=MasterMode  countermode=CounterMode  init=Init  commands=Runtime  term=Term  ts=Ts  pciSlot=pciSlot
  Product : Product  SaturateOnIntegerOverflow=on  InputSameDT=on
  Product1 : Product  Inputs=/  SaturateOnIntegerOverflow=on  InputSameDT=on
  Relational Operator : RelationalOperator  Operator=<  InputSameDT=on
  Relational Operator1 : RelationalOperator  Operator=>  InputSameDT=on
  Saturation : Saturate  UpperLimit=duty/2  LowerLimit=duty/(2^16-1)  ZeroCross=off
  Saturation1 : Saturate  UpperLimit=(1-duty)/2  LowerLimit=(1-duty)/(2^16-1)  ZeroCross=off
  Sum : Sum  Inputs=-+  SaturateOnIntegerOverflow=on  InputSameDT=on
  Sum4 : Sum  Inputs=+-  SaturateOnIntegerOverflow=on  InputSameDT=on
  Switch1 : Switch  Threshold=0.5  InputSameDT=on
  Switch2 : Switch  Threshold=0.5  InputSameDT=on
  Unit Delay2 : UnitDelay  X0=2  SampleTime=Ts
  arm : Constant
  duty : Constant  Value=duty
  level : Constant  Value=level
  seq : Constant  Value=seq
  wires:
  Data Type Conversion5/1 -> Logical Operator1/1
  Data Type Conversion3/1 -> Combinatorial  Logic/1
  Data Type Conversion2/1 -> Demux/1
  Data Type Conversion1/1 -> Mux1/3, Mux/1
  Data Type Conversion4/1 -> Mux1/2, Mux/2
  1/relFreq1/1 -> Relational Operator/2
  Product/1 -> Sum/1, Switch1/3, Switch2/1
  1/relFreq2/1 -> Relational Operator1/2
  Relational Operator1/1 -> Data Type Conversion1/1
  Relational Operator/1 -> Data Type Conversion4/1
  Combinatorial  Logic/1 -> Logical Operator/2
  Logical Operator/1 -> Data Type Conversion2/1
  Unit Delay2/1 -> Sum4/2
  Sum4/1 -> Abs/1
  Logical Operator1/1 -> Logical Operator/1
  Demux/1 -> "PCI-CTR05  "/3
  Demux/2 -> "PCI-CTR05  "/4
  Demux/3 -> "PCI-CTR05  "/5
  Demux/4 -> "PCI-CTR05  "/6
  level/1 -> Mux/4
  Switch1/1 -> "PCI-CTR05  "/1
  Switch2/1 -> "PCI-CTR05  "/2
  seq/1 -> Switch1/2, Switch2/2, Mux/5
  Sum/1 -> Switch1/1, Switch2/3
  Saturation/1 -> Saturation1/1
  f/1 -> Saturation/1
  Mux1/1 -> Sum4/1, Unit Delay2/1
  arm/1 -> Mux1/1, Mux/3
  Abs/1 -> Data Type Conversion5/1
  Mux/1 -> Data Type Conversion3/1
  Saturation1/1 -> Product1/1, Relational Operator1/1, Relational Operator/1
  duty/1 -> Product/1
  Product1/1 -> Product/2, Sum/2

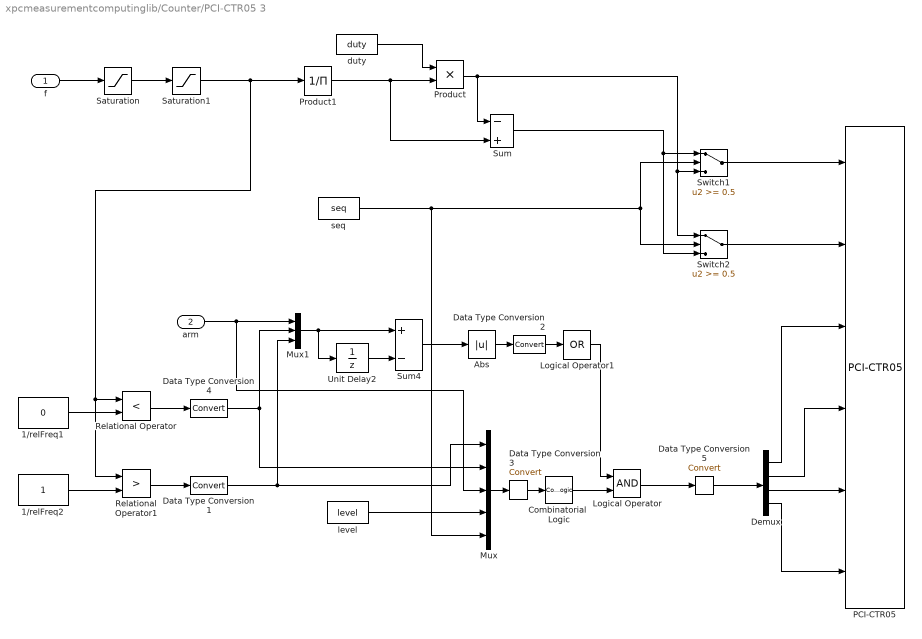
== system xpcmeasurementcomputinglib/Counter/PCI-CTR05 3 ==
  f : Inport  LatchInput=off
  arm : Inport  Port=2  LatchInput=off
  1/relFreq1 : Constant  Value=0
  1/relFreq2 : Constant
  Abs : Abs  SaturateOnIntegerOverflow=on
  Combinatorial  Logic : CombinatorialLogic  TruthTable=[0,0,1,0;0,0,1,0;0,0,0,1;0,0,0,1;0,1,0,0;1,0,0,0;0,1,0,0;1,0,0,0;0,0,1,0;0,0,1,0;0,0,0,1;0,0,0,1;0,0,1,0;0,0,1,0;0,0,1,0;0,0,1,0;0,0,1,0;0,0,1,0;0,0,0,1;0,0,0,1;0,0,0,1;0,0,0,1;0,0,0,1;0,0,0,1;0,0,0,0;0,0,0,0;0,0,0,0;0,0,0,0;0,0,0,0;0,0,0,0;0,0,0,0;0,0,0,0]
  Data Type Conversion1 : DataTypeConversion  OutDataTypeMode=double  SaturateOnIntegerOverflow=on  RndMeth=Zero
  Data Type Conversion2 : DataTypeConversion  SaturateOnIntegerOverflow=on  RndMeth=Zero
  Data Type Conversion3 : DataTypeConversion  SaturateOnIntegerOverflow=on  RndMeth=Zero
  Data Type Conversion4 : DataTypeConversion  OutDataTypeMode=double  SaturateOnIntegerOverflow=on  RndMeth=Zero
  Data Type Conversion5 : DataTypeConversion  SaturateOnIntegerOverflow=on  RndMeth=Zero
  Demux : Demux
  Logical Operator : Logic
  Logical Operator1 : Logic  Operator=OR  Inputs=1
  Mux : Mux  Inputs=5
  Mux1 : Mux  Inputs=3
  "PCI-CTR05  " : xpcmeasurementcomputinglib/Counter/PCI-CTR05    mastermode=MasterMode  countermode=CounterMode  init=Init  commands=Runtime  term=Term  ts=Ts  pciSlot=pciSlot
  Product : Product  SaturateOnIntegerOverflow=on  InputSameDT=on
  Product1 : Product  Inputs=/  SaturateOnIntegerOverflow=on  InputSameDT=on
  Relational Operator : RelationalOperator  Operator=<  InputSameDT=on
  Relational Operator1 : RelationalOperator  Operator=>  InputSameDT=on
  Saturation : Saturate  UpperLimit=duty/2  LowerLimit=duty/(2^16-1)  ZeroCross=off
  Saturation1 : Saturate  UpperLimit=(1-duty)/2  LowerLimit=(1-duty)/(2^16-1)  ZeroCross=off
  Sum : Sum  Inputs=-+  SaturateOnIntegerOverflow=on  InputSameDT=on
  Sum4 : Sum  Inputs=+-  SaturateOnIntegerOverflow=on  InputSameDT=on
  Switch1 : Switch  Threshold=0.5  InputSameDT=on
  Switch2 : Switch  Threshold=0.5  InputSameDT=on
  Unit Delay2 : UnitDelay  X0=2  SampleTime=Ts
  duty : Constant  Value=duty
  level : Constant  Value=level
  seq : Constant  Value=seq
  wires:
  Data Type Conversion5/1 -> Demux/1
  Data Type Conversion3/1 -> Combinatorial  Logic/1
  Data Type Conversion2/1 -> Logical Operator1/1
  Data Type Conversion1/1 -> Mux1/3, Mux/1
  Data Type Conversion4/1 -> Mux1/2, Mux/2
  1/relFreq1/1 -> Relational Operator/2
  Product/1 -> Sum/1, Switch1/3, Switch2/1
  1/relFreq2/1 -> Relational Operator1/2
  Relational Operator1/1 -> Data Type Conversion1/1
  Relational Operator/1 -> Data Type Conversion4/1
  Combinatorial  Logic/1 -> Logical Operator/2
  Logical Operator/1 -> Data Type Conversion5/1
  Unit Delay2/1 -> Sum4/2
  Sum4/1 -> Abs/1
  Logical Operator1/1 -> Logical Operator/1
  Demux/1 -> "PCI-CTR05  "/3
  Demux/2 -> "PCI-CTR05  "/4
  Demux/3 -> "PCI-CTR05  "/5
  Demux/4 -> "PCI-CTR05  "/6
  level/1 -> Mux/4
  Switch1/1 -> "PCI-CTR05  "/1
  Switch2/1 -> "PCI-CTR05  "/2
  seq/1 -> Switch1/2, Switch2/2, Mux/5
  Sum/1 -> Switch1/1, Switch2/3
  Saturation/1 -> Saturation1/1
  f/1 -> Saturation/1
  Mux1/1 -> Sum4/1, Unit Delay2/1
  arm/1 -> Mux1/1, Mux/3
  Abs/1 -> Data Type Conversion2/1
  Mux/1 -> Data Type Conversion3/1
  Saturation1/1 -> Product1/1, Relational Operator1/1, Relational Operator/1
  duty/1 -> Product/1
  Product1/1 -> Product/2, Sum/2

== system xpcmeasurementcomputinglib/Counter/PCI-CTR05 4 ==
  Demux : Demux  Outputs=2
  "PCI-CTR05  " : xpcmeasurementcomputinglib/Counter/PCI-CTR05    mastermode=MasterMode  countermode=CounterMode  init=Init  commands=Runtime  term=Term  ts=Ts  pciSlot=pciSlot
  Product : Product  Inputs=/  SaturateOnIntegerOverflow=on  InputSameDT=on
  Product1 : Product  Inputs=**  SaturateOnIntegerOverflow=on  InputSameDT=on
  f : Outport
  dc : Outport  Port=2
  wires:
  "PCI-CTR05  "/1 -> Demux/1
  Product1/1 -> dc/1
  Product/1 -> Product1/2, f/1
  Demux/2 -> Product/1
  Demux/1 -> Product1/1

== system xpcmeasurementcomputinglib/Counter/PCI-CTR05 5 ==
  "PCI-CTR05  " : xpcmeasurementcomputinglib/Counter/PCI-CTR05    mastermode=MasterMode  countermode=CounterMode  init=Init  commands=Runtime  term=Term  ts=Ts  pciSlot=pciSlot
  Product : Product  Inputs=/  SaturateOnIntegerOverflow=on  InputSameDT=on
  f : Outport
  wires:
  Product/1 -> f/1
  "PCI-CTR05  "/1 -> Product/1

== system xpcmeasurementcomputinglib/Digital Input/CIO-PDISO16  ==
  DAC1 : S-Function  FunctionName=dicbpdiso16  Parameters=n_channels,port,sample_time,baseaddress
  out_1 : Outport  InitialOutput=0
  wires:
  DAC1/1 -> out_1/1

== system xpcmeasurementcomputinglib/Digital Input/PC104-DAS16JR 12  ==
  DAC1 : S-Function  FunctionName=dicbpc104das16jr  Parameters=n_channels,sample_time,baseaddress
  out_1 : Outport  InitialOutput=0
  wires:
  DAC1/1 -> out_1/1

== system xpcmeasurementcomputinglib/Digital Input/PC104-DAS16JR 16  ==
  DAC1 : S-Function  FunctionName=dicbpc104das16jr  Parameters=n_channels,sample_time,baseaddress
  out_1 : Outport  InitialOutput=0
  wires:
  DAC1/1 -> out_1/1

== system xpcmeasurementcomputinglib/Digital Output/CIO-DO24DD  ==
  in_1 : Inport  LatchInput=off
  DAC : S-Function  FunctionName=docbciodo24dd  Parameters=n_channels,port,sample_time,baseaddress
  wires:
  in_1/1 -> DAC/1

== system xpcmeasurementcomputinglib/Digital Output/CIO-PDISO16  ==
  in_1 : Inport  LatchInput=off
  DAC : S-Function  FunctionName=docbpdiso16  Parameters=n_channels,port,sample_time,baseaddress
  wires:
  in_1/1 -> DAC/1

== system xpcmeasurementcomputinglib/Digital Output/PC104-DAS16JR 12  ==
  in_1 : Inport  LatchInput=off
  DAC : S-Function  FunctionName=docbpc104das16jr  Parameters=n_channels,sample_time,baseaddress
  wires:
  in_1/1 -> DAC/1

== system xpcmeasurementcomputinglib/Digital Output/PC104-DAS16JR 16  ==
  in_1 : Inport  LatchInput=off
  DAC : S-Function  FunctionName=docbpc104das16jr  Parameters=n_channels,sample_time,baseaddress
  wires:
  in_1/1 -> DAC/1
